simulink model "cycleswitching"  (R2018a)
settings: Solver=VariableStepAuto  StartTime=0.0  StopTime=0.5  RelTol=1e-3
libraries: powerlib x26, simulink x4
settings Model: Creator=DaniShah  LastModifiedBy=DaniShah

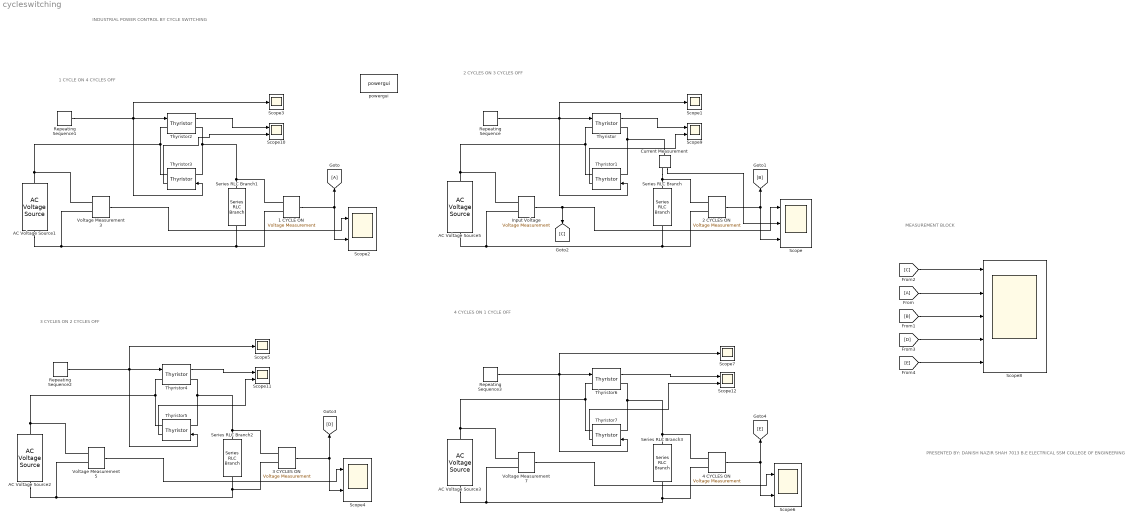
== system cycleswitching ==
  note: MEASUREMENT BLOCK
  note: PRESENTED BY:
      | DANISH NAZIR SHAH
      | 7013 B.E ELECTRICAL
      | SSM COLLEGE OF ENGINEERING
  note: INDUSTRIAL POWER CONTROL BY CYCLE SWITCHING
  note: 1 CYCLE ON 4 CYCLES OFF
  note: 2 CYCLES ON 3 CYCLES OFF
  note: 3 CYCLES ON 2 CYCLES OFF
  note: 4 CYCLES ON 1 CYCLE OFF
  1 CYCLE ON : powerlib/Measurements/Voltage Measurement  PhasorSimulation=off  OutputType=Complex  PSBequivalent=0
  2 CYCLES ON : powerlib/Measurements/Voltage Measurement  PhasorSimulation=off  OutputType=Complex  PSBequivalent=0
  3 CYCLES ON : powerlib/Measurements/Voltage Measurement  PhasorSimulation=off  OutputType=Complex  PSBequivalent=0
  4 CYCLES ON : powerlib/Measurements/Voltage Measurement  PhasorSimulation=off  OutputType=Complex  PSBequivalent=0
  AC Voltage Source{1..3,5} (4 alike) : powerlib/Electrical Sources/AC Voltage Source  Amplitude=230  Phase=0  Frequency=50  SampleTime=0  Measurements=None  BusType=swing  Pref=10e3  Qref=0  Qmin=-inf  Qmax=+inf
  Current Measurement : powerlib/Measurements/Current Measurement  PhasorSimulation=off  OutputType=Complex  PSBequivalent=0
  Input Voltage : powerlib/Measurements/Voltage Measurement  PhasorSimulation=off  OutputType=Complex  PSBequivalent=0
  Repeating Sequence : simulink/Sources/Repeating Sequence  rep_seq_t=[0 0+eps 0.04 0.04+eps 0.1 0.1+eps]  rep_seq_y=[0 1 1 0 0 1]
  Repeating Sequence1 : simulink/Sources/Repeating Sequence  rep_seq_t=[0 0+eps 0.02 0.02+eps 0.1 0.1+eps]  rep_seq_y=[0 1 1 0 0 1]
  Repeating Sequence2 : simulink/Sources/Repeating Sequence  rep_seq_t=[0 0+eps 0.06 0.06+eps 0.1 0.1+eps]  rep_seq_y=[0 1 1 0 0 1]
  Repeating Sequence3 : simulink/Sources/Repeating Sequence  rep_seq_t=[0 0+eps 0.08 0.08+eps 0.1 0.1+eps]  rep_seq_y=[0 1 1 0 0 1]
  Scope : Scope  NumInputPorts=3
  Scope{1,3,5,7} (4 alike) : Scope
  Scope{2,4,6,9..12} (7 alike) : Scope  NumInputPorts=2
  Scope8 : Scope  NumInputPorts=5
  Series RLC Branch : powerlib/Elements/Series RLC Branch  LConnTagsString=__new0  RConnTagsString=__new0  BranchType=R  Resistance=46  Inductance=10  SetiL0=off  InitialCurrent=0  Capacitance=10  Setx0=off  InitialVoltage=0  Measurements=None
  Series RLC Branch1 : powerlib/Elements/Series RLC Branch  LConnTagsString=__new0  RConnTagsString=__new0  BranchType=R  Resistance=46  Inductance=2  SetiL0=off  InitialCurrent=0  Capacitance=2  Setx0=off  InitialVoltage=0  Measurements=None
  Series RLC Branch2 : powerlib/Elements/Series RLC Branch  LConnTagsString=__new0  RConnTagsString=__new0  BranchType=R  Resistance=46  Inductance=1e-3  SetiL0=off  InitialCurrent=0  Capacitance=1e-6  Setx0=off  InitialVoltage=0  Measurements=None
  Series RLC Branch3 : powerlib/Elements/Series RLC Branch  LConnTagsString=__new0  RConnTagsString=__new0  BranchType=R  Resistance=46  Inductance=1e-3  SetiL0=off  InitialCurrent=0  Capacitance=1e-6  Setx0=off  InitialVoltage=0  Measurements=None
  Thyristor{,1..7} (8 alike) : powerlib/Power Electronics/Thyristor  Ron=0.001  Lon=0  Vf=0.8  IC=0  Rs=500  Cs=250e-9  Measurements=on
  Voltage Measurement3 : powerlib/Measurements/Voltage Measurement  PhasorSimulation=off  OutputType=Complex  PSBequivalent=0
  Voltage Measurement5 : powerlib/Measurements/Voltage Measurement  PhasorSimulation=off  OutputType=Complex  PSBequivalent=0
  Voltage Measurement7 : powerlib/Measurements/Voltage Measurement  PhasorSimulation=off  OutputType=Complex  PSBequivalent=0
  powergui : powerlib/powergui  Priority=1  SimulationMode=Continuous  SampleTime=50e-6  frequency=60  Iterations=50  frequencyindice=50  Pbase=100e6  ErrMax=1e-4  UnitsV=kV  UnitsW=MW  buscounter=0  FunctionMessages=off  echomessages=off  EnableUseOfTLC=off  CurrentSourceSwitches=off  DisableSnubberDevices=off  DisableRonSwitches=off  DisableVfSwitches=off  DisplayEquations=off  SolverType=Tustin/Backward Euler (TBE)  Interpol=off  ExternalGateDelay=off  methode=off  Ts=100  x0status=blocks  SPID=on  SwTol=0  HookPort=off  RestoreLinks=warning  ResistiveCurrentMeasurement=off  Frange=[0:2:500]  Ylog=off  Xlog=on  ShowGrid=off  save=off  variable=ZData  structure=ScopeData2  ZoomFFT=off  StartTime=0.0  cycles=2  DisplayStyle=1  fundamental=50  FreqAxis=on  MaxFrequency=500  frequencyindicesteady=1  RmsSteady=1  display=off
  wires:
  Input Voltage/1 -> [C], Scope/1
  Repeating Sequence/1 -> Scope1/1, Thyristor/1, Thyristor1/1
  Repeating Sequence1/1 -> Thyristor3/1, Thyristor2/1, Scope3/1
  Voltage Measurement3/1 -> Scope2/1
  1 CYCLE ON/1 -> Scope2/2, [A]
  3 CYCLES ON/1 -> [D], Scope4/2
  Voltage Measurement5/1 -> Scope4/1
  Repeating Sequence2/1 -> Scope5/1, Thyristor4/1, Thyristor5/1
  Repeating Sequence3/1 -> Thyristor7/1, Thyristor6/1, Scope7/1
  Voltage Measurement7/1 -> Scope6/1
  4 CYCLES ON/1 -> [E], Scope6/2
  2 CYCLES ON/1 -> Scope/3, [B]
  [A] -> Scope8/2
  [B] -> Scope8/3
  [C] -> Scope8/1
  [D] -> Scope8/4
  [E] -> Scope8/5
  Thyristor/1 -> Scope9/1
  Thyristor1/1 -> Scope9/2
  Current Measurement/1 -> Scope/2
  Thyristor2/1 -> Scope10/1
  Thyristor3/1 -> Scope10/2
  Thyristor4/1 -> Scope11/1
  Thyristor5/1 -> Scope11/2
  Thyristor6/1 -> Scope12/1
  Thyristor7/1 -> Scope12/2
  connections:
  Thyristor1/LConn1 -- Thyristor/RConn1 -- Current Measurement/LConn1
  Thyristor/LConn1 -- AC Voltage Source5/RConn1 -- Input Voltage/LConn1 -- Thyristor1/RConn1
  Input Voltage/LConn2 -- AC Voltage Source5/LConn1 -- 2 CYCLES ON/LConn2 -- Series RLC Branch/RConn1
  1 CYCLE ON/LConn1 -- Series RLC Branch1/LConn1 -- Thyristor3/LConn1 -- Thyristor2/RConn1
  Voltage Measurement3/LConn1 -- AC Voltage Source1/RConn1 -- Thyristor2/LConn1 -- Thyristor3/RConn1
  Voltage Measurement3/LConn2 -- AC Voltage Source1/LConn1 -- Series RLC Branch1/RConn1 -- 1 CYCLE ON/LConn2
  Series RLC Branch2/LConn1 -- Thyristor4/RConn1 -- Thyristor5/LConn1 -- 3 CYCLES ON/LConn1
  AC Voltage Source2/RConn1 -- Thyristor5/RConn1 -- Thyristor4/LConn1 -- Voltage Measurement5/LConn1
  Series RLC Branch2/RConn1 -- Voltage Measurement5/LConn2 -- AC Voltage Source2/LConn1 -- 3 CYCLES ON/LConn2
  Thyristor6/RConn1 -- Series RLC Branch3/LConn1 -- 4 CYCLES ON/LConn1 -- Thyristor7/LConn1
  Thyristor7/RConn1 -- AC Voltage Source3/RConn1 -- Voltage Measurement7/LConn1 -- Thyristor6/LConn1
  Voltage Measurement7/LConn2 -- Series RLC Branch3/RConn1 -- 4 CYCLES ON/LConn2 -- AC Voltage Source3/LConn1
  Series RLC Branch/LConn1 -- Current Measurement/RConn1 -- 2 CYCLES ON/LConn1
